simulink model "piregulator"  (R2015a)
settings: Solver=ode45  StartTime=0.0  StopTime=10.0  RelTol=1e-3
undefined symbols (not defined in the file): K_i, K_p
settings Model: CovSFcnEnable=off  Creator=Heath  LastModifiedBy=Hofmann
settings DebuggingCC: UnderspecifiedInitializationDetection=Classic  MergeDetectMultiDrivingBlocksExec=none  SolverPrmCheckMsg=warning  StateNameClashWarn=warning

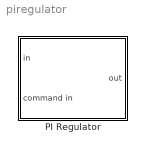
== system piregulator ==
  PI Regulator : Subsystem

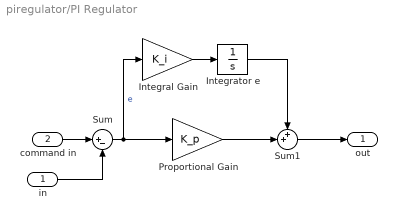
== system piregulator/PI Regulator ==
  in : Inport
  command in : Inport  Port=2
  Integral Gain : Gain  Gain=K_i  SaturateOnIntegerOverflow=on  OutDataTypeStr=Inherit: Same as input  ParamDataTypeStr=Inherit: Same as input
  Integrator e : Integrator
  Proportional Gain : Gain  Gain=K_p  SaturateOnIntegerOverflow=on  OutDataTypeStr=Inherit: Same as input  ParamDataTypeStr=Inherit: Same as input
  Sum : Sum  Inputs=|+-  SaturateOnIntegerOverflow=on
  Sum1 : Sum  Inputs=++|  SaturateOnIntegerOverflow=on
  out : Outport
  wires:
  Sum/1 -> Integral Gain/1, Proportional Gain/1  "e"
  command in/1 -> Sum/1
  in/1 -> Sum/2
  Proportional Gain/1 -> Sum1/2
  Sum1/1 -> out/1
  Integral Gain/1 -> Integrator e/1
  Integrator e/1 -> Sum1/1
